simulink library "limblab"  (Simulink 8.0)
settings: Solver=ode45  SolverMode=SingleTasking  StartTime=0.0  StopTime=10.0  RelTol=1e-3
undefined symbols (not defined in the file or in its folder): dfilt, DiscIntNeverNeededParam
libraries: simulink x25, xpclib x10, limblab x9, xpcnilib x5, dsparch4 x4, dspsigops x2, xpcmeasurementcomputinglib x2, dspmtrx3 x1, simulink_extras x1
(part 1 of 2)
settings Model: Creator=limblab  LastModifiedBy=system administrator

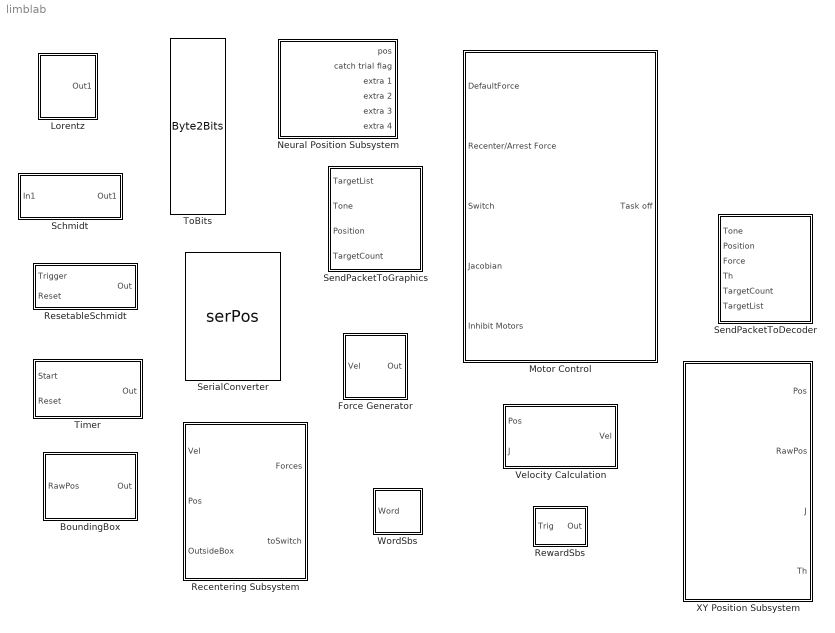
== system limblab ==
  BoundingBox : Subsystem
  Force Generator : Subsystem
  Lorentz : Subsystem  mask(Lorentz attractor){y0=.1}
      mask prompts: y0 "Initial Condition"
      mask help: Creats chaotic oscelations using a lorentz attractor algorithm.
      mask Help:
      | Creats chaotic oscelations using a lorentz attractor algorithm.
      | 
      | This particular oscilator has the parameters:
      | rho = 28
      | beta = 8/3
      | sigma = 10
      | 
      | The initial condition y0 can be specified as a parameter.
      | 
      | Other initial conditions (x0 and z0) are 0.1.
      mask Display: port_label('output', 1, 'Out')
  Motor Control : Subsystem
  Neural Position Subsystem : Subsystem  SystemSampleTime=0.01  mask(Neural Position Subsystem){}
      mask help: Uses a UDP receive block to receive and parse the sent neural position from the real time system.
      mask Display:
      | port_label('output',1,'pos')
      | port_label('output',2,'catch trial flag')
      | port_label('output',3,'extra 1')
      | port_label('output',4,'extra 2')
      | port_label('output',5,'extra 3')
      | port_label('output',6,'extra 4')
  Recentering Subsystem : Subsystem
  ResetableSchmidt : Subsystem  mask{Time=3}
  RewardSbs : Subsystem
  Schmidt : Subsystem  mask(Schmidt Trigger){Time=.3}
      mask help: Creates an output pulse of the specified time in seconds when trig goes high
      mask Help: Creates an output pulse of the specified time in seconds when trig goes high
      mask Display:
      | port_label('output',1,'out')
      | port_label('input',1,'trig')
      | fprintf('t = %.2f',Time)
  SendPacketToDecoder : Subsystem
  SendPacketToGraphics : Subsystem
  SerialConverter : S-Function  FunctionName=serPos  EnableBusSupport=off
      mask Display:
      | port_label('output', 1, 'Byte Out')
      | port_label('input', 1, 'index')
      | port_label('input', 2, 'sh')
      | port_label('input', 3, 'el')
  Timer : Subsystem  mask{Time=.1}
      mask prompts: Time "Timeout"
      mask Display:
      | port_label('output',1,'out')
      | port_label('input',1,'start')
      | port_label('input',2,'reset')
      | fprintf('t = %.2f',Time)
  ToBits : S-Function  FunctionName=Byte2Bits  EnableBusSupport=off
      mask Display:
      | port_label('input', 1, 'u')
      | port_label('output', 1, 'y0')
      | port_label('output', 2, 'y1')
      | port_label('output', 3, 'y2')
      | port_label('output', 4, 'y3')
      | port_label('output', 5, 'y4')
      | port_label('output', 6, 'y5')
      | port_label('output', 7, 'y6')
      | port_label('output', 8, 'y7')
  Velocity Calculation : Subsystem
  WordSbs : Subsystem
  XY Position Subsystem : Subsystem

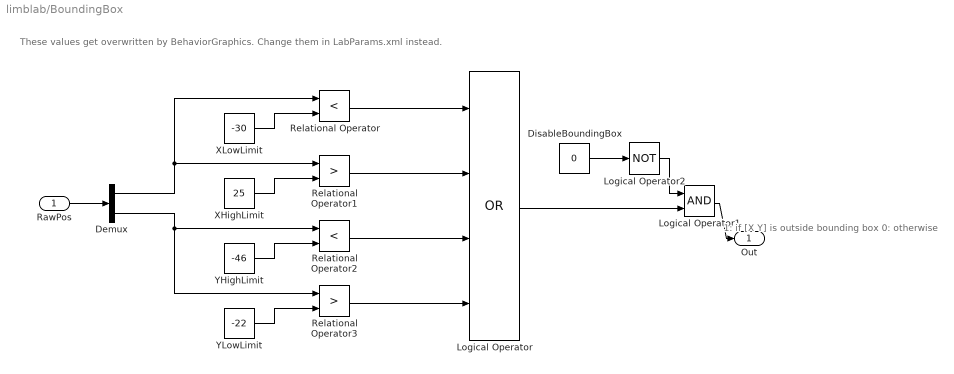
== system limblab/BoundingBox ==
  note: These values get overwritten by BehaviorGraphics. Change them in LabParams.xml instead.
  note: 1: if [X Y] is outside
      | bounding box
      | 0: otherwise
  RawPos : Inport
  Demux : Demux  Outputs=2
  DisableBoundingBox : Constant  Value=0
  Logical Operator : Logic  Operator=OR  Inputs=4  AllPortsSameDT=off  OutDataTypeStr=boolean
  Logical Operator1 : Logic  AllPortsSameDT=off  OutDataTypeStr=boolean
  Logical Operator2 : Logic  Operator=NOT  AllPortsSameDT=off  OutDataTypeStr=boolean
  Relational Operator : RelationalOperator  Operator=<  OutDataTypeStr=boolean
  Relational Operator1 : RelationalOperator  Operator=>  OutDataTypeStr=boolean
  Relational Operator2 : RelationalOperator  Operator=<  OutDataTypeStr=boolean
  Relational Operator3 : RelationalOperator  Operator=>  OutDataTypeStr=boolean
  XHighLimit : Constant  Value=25
  XLowLimit : Constant  Value=-30
  YHighLimit : Constant  Value=-46
  YLowLimit : Constant  Value=-22
  Out : Outport
  wires:
  XLowLimit/1 -> Relational Operator/2
  XHighLimit/1 -> Relational Operator1/2
  YHighLimit/1 -> Relational Operator2/2
  YLowLimit/1 -> Relational Operator3/2
  Relational Operator/1 -> Logical Operator/1
  Relational Operator1/1 -> Logical Operator/2
  Relational Operator2/1 -> Logical Operator/3
  Relational Operator3/1 -> Logical Operator/4
  RawPos/1 -> Demux/1
  Demux/1 -> Relational Operator/1, Relational Operator1/1
  Demux/2 -> Relational Operator2/1, Relational Operator3/1
  Logical Operator1/1 -> Out/1
  Logical Operator/1 -> Logical Operator1/2
  DisableBoundingBox/1 -> Logical Operator2/1
  Logical Operator2/1 -> Logical Operator1/1

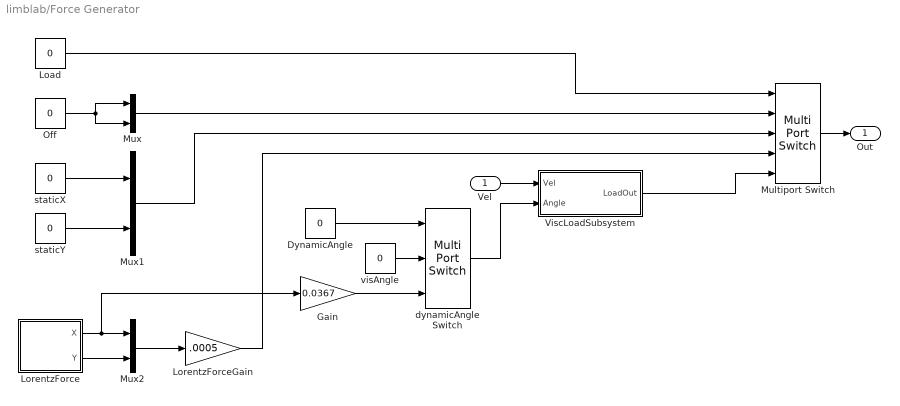
== system limblab/Force Generator ==
  Vel : Inport
  DynamicAngle : Constant  Value=0
  Gain : Gain  Gain=0.0367
  Load : Constant  Value=0
  LorentzForce : Subsystem
  LorentzForceGain : Gain  Gain=.0005
  Multiport Switch : MultiPortSwitch  DataPortOrder=Zero-based contiguous  Inputs=4  zeroidx=on
  Mux : Mux  Inputs=2
  Mux1 : Mux  Inputs=2
  Mux2 : Mux  Inputs=2
  Off : Constant  Value=0
  ViscLoadSubsystem : Subsystem
  dynamicAngle Switch : MultiPortSwitch  DataPortOrder=Zero-based contiguous  Inputs=2  zeroidx=on
  staticX : Constant  Value=0
  staticY : Constant  Value=0
  visAngle : Constant  Value=0
  Out : Outport
  wires:
  Off/1 -> Mux/2, Mux/1
  Multiport Switch/1 -> Out/1
  Mux/1 -> Multiport Switch/2
  Load/1 -> Multiport Switch/1
  Mux1/1 -> Multiport Switch/3
  staticX/1 -> Mux1/1
  staticY/1 -> Mux1/2
  LorentzForce/1(X) -> Mux2/1, Gain/1
  LorentzForce/2(Y) -> Mux2/2
  Mux2/1 -> LorentzForceGain/1
  LorentzForceGain/1 -> Multiport Switch/4
  Vel/1 -> ViscLoadSubsystem/1(Vel)
  ViscLoadSubsystem/1(LoadOut) -> Multiport Switch/5
  visAngle/1 -> dynamicAngle Switch/2
  DynamicAngle/1 -> dynamicAngle Switch/1
  dynamicAngle Switch/1 -> ViscLoadSubsystem/2(Angle)
  Gain/1 -> dynamicAngle Switch/3

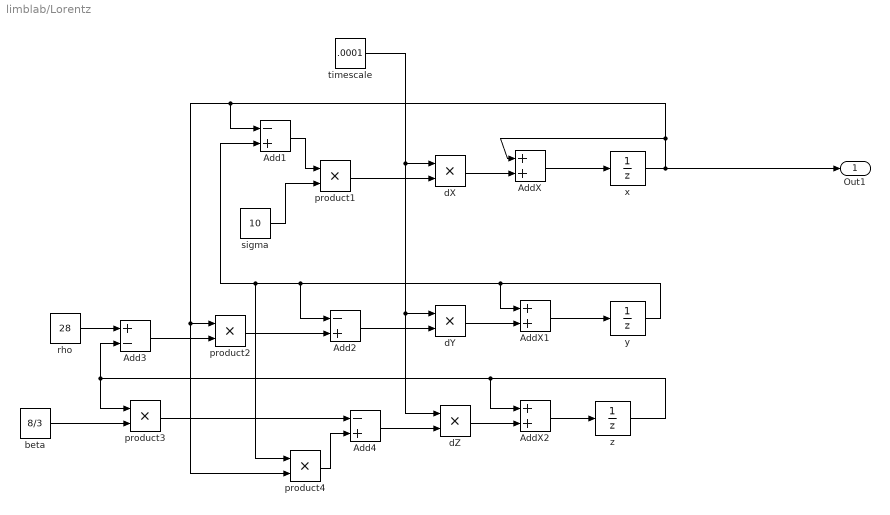
== system limblab/Lorentz ==
  Add1 : Sum  Inputs=-+
  Add2 : Sum  Inputs=-+
  Add3 : Sum  Inputs=+-
  Add4 : Sum  Inputs=-+
  AddX : Sum
  AddX1 : Sum
  AddX2 : Sum
  beta : Constant  Value=8/3
  dX : Product  RndMeth=Zero
  dY : Product  RndMeth=Zero
  dZ : Product  RndMeth=Zero
  product{1..4} (4 alike) : Product  RndMeth=Zero
  rho : Constant  Value=28
  sigma : Constant  Value=10
  timescale : Constant  Value=.0001
  x : UnitDelay  InitialCondition=.1  SampleTime=.001
  y : UnitDelay  InitialCondition=y0  SampleTime=.001
  z : UnitDelay  InitialCondition=.1  SampleTime=.001
  Out1 : Outport
  wires:
  AddX/1 -> x/1
  AddX1/1 -> y/1
  AddX2/1 -> z/1
  y/1 -> AddX1/1, Add2/1, Add1/2, product4/1
  z/1 -> AddX2/1, Add3/2, product3/1
  x/1 -> Out1/1, AddX/1, Add1/1, product2/1, product4/2
  dX/1 -> AddX/2
  dY/1 -> AddX1/2
  dZ/1 -> AddX2/2
  timescale/1 -> dX/1, dY/1, dZ/1
  sigma/1 -> product1/2
  product1/1 -> dX/2
  Add1/1 -> product1/1
  Add2/1 -> dY/2
  product2/1 -> Add2/2
  Add3/1 -> product2/2
  rho/1 -> Add3/1
  beta/1 -> product3/2
  product3/1 -> Add4/1
  product4/1 -> Add4/2
  Add4/1 -> dZ/2

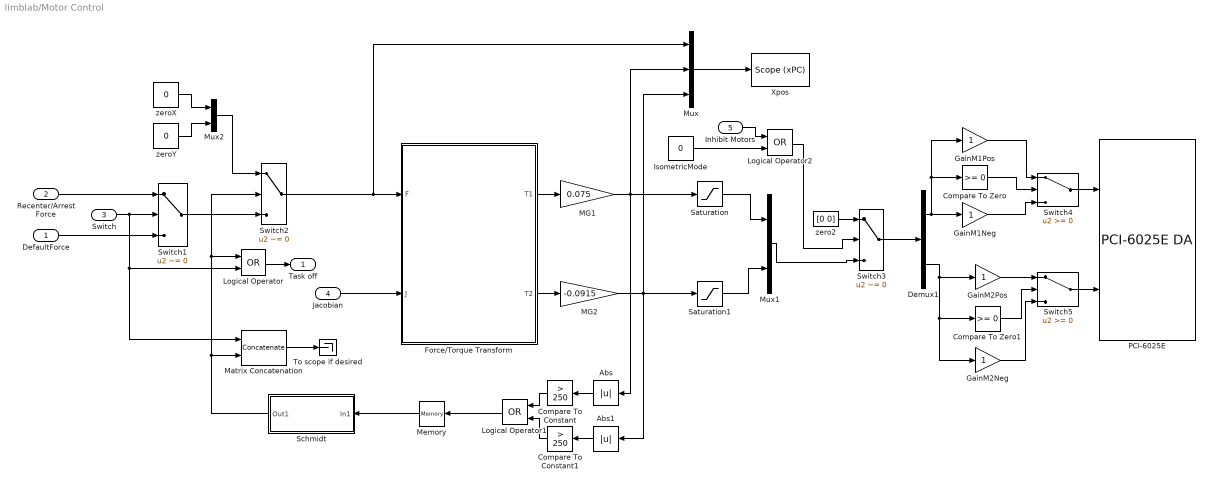
== system limblab/Motor Control ==
  DefaultForce : Inport
  Recenter/Arrest Force : Inport  Port=2
  Switch : Inport  Port=3
  Jacobian : Inport  Port=4
  Inhibit Motors : Inport  Port=5
  Abs : Abs
  Abs1 : Abs
  Compare To Constant : simulink/Logic and Bit Operations/Compare To Constant  relop=>  const=250  OutDataTypeStr=uint8  ZeroCross=off
  Compare To Constant1 : simulink/Logic and Bit Operations/Compare To Constant  relop=>  const=250  OutDataTypeStr=uint8  ZeroCross=off
  Compare To Zero : simulink/Logic and Bit Operations/Compare To Zero  relop=>=  OutDataTypeStr=boolean
  Compare To Zero1 : simulink/Logic and Bit Operations/Compare To Zero  relop=>=  OutDataTypeStr=boolean
  Demux1 : Demux  Outputs=2
  Force/Torque Transform : Subsystem  TreatAsAtomicUnit=on
  GainM1Neg : Gain
  GainM1Pos : Gain
  GainM2Neg : Gain
  GainM2Pos : Gain
  IsometricMode : Constant  Value=0
  Logical Operator1 : Logic  Operator=OR  AllPortsSameDT=off  OutDataTypeStr=boolean
  Logical Operator : Logic  Operator=OR  AllPortsSameDT=off  OutDataTypeStr=boolean
  Logical Operator2 : Logic  Operator=OR  AllPortsSameDT=off  OutDataTypeStr=boolean
  MG1 : Gain  Gain=0.075
  MG2 : Gain  Gain=-0.0915
  Matrix Concatenation : Concatenate
  Memory : Memory
  Mux : Mux  Inputs=3
  Mux1 : Mux  Inputs=2
  Mux2 : Mux  Inputs=2
  "PCI-6025E " : xpcnilib/D//A/E Series/PCI-6025E DA  channel=[1 2]  reset=[1 1]  initValue=[0 0]  sampletime=0.001  slot=-1
  Saturation : Saturate  UpperLimit=7.5  LowerLimit=-7.5
  Saturation1 : Saturate  UpperLimit=7.5  LowerLimit=-7.5
  Schmidt : Subsystem  mask(Schmidt Trigger){Time=10}
      mask help: Creates an output pulse of the specified time in seconds when trig goes high
      mask Help: Creates an output pulse of the specified time in seconds when trig goes high
      mask Display:
      | port_label('output',1,'out')
      | port_label('input',1,'trig')
      | fprintf('t = %d',Time)
  Switch1 : Switch  Criteria=u2 ~= 0  ZeroCross=off
  Switch2 : Switch  Criteria=u2 ~= 0  ZeroCross=off
  Switch3 : Switch  Criteria=u2 ~= 0  ZeroCross=off
  Switch4 : Switch
  Switch5 : Switch
  To scope if desired : Terminator
  Xpos : xpclib/Misc./Scope (xPC)   scopeno=4  scopetype=Target  autostart=on  viewmode=Numerical  formatstr='%15.2f Fx,%15.2f Fy,%15.2f T1,%15.2f T2'  grid=on  ylimits=[-10,10]  nosamples=10  noprepostsamples=0  interleave=10  triggermode=FreeRun  triggersignal=1  triggerlevel=0.0  triggerslope=Either  triggerscope=1  triggersample=0  filename=data.dat  mode=Lazy  writesize=512  autorestart=off  dynamicfilemode=off  maxwritefilesize=512*1024^2
  zero2 : Constant  Value=[0 0]
  zeroX : Constant  Value=0
  zeroY : Constant  Value=0
  Task off : Outport
  wires:
  MG1/1 -> Abs/1, Saturation/1, Mux/2
  MG2/1 -> Abs1/1, Saturation1/1, Mux/3
  Force/Torque Transform/1(T1) -> MG1/1
  Force/Torque Transform/2(T2) -> MG2/1
  zeroX/1 -> Mux2/1
  zeroY/1 -> Mux2/2
  Mux2/1 -> Switch2/1
  Switch1/1 -> Switch2/3
  Switch2/1 -> Force/Torque Transform/1(F), Mux/1
  Schmidt/1(Out1) -> Logical Operator/1, Switch2/2, Matrix Concatenation/2
  Compare To Constant/1 -> Logical Operator1/1
  Compare To Constant1/1 -> Logical Operator1/2
  Memory/1 -> Schmidt/1(In1)
  Logical Operator1/1 -> Memory/1
  Matrix Concatenation/1 -> To scope if desired/1
  Jacobian/1 -> Force/Torque Transform/2(J)
  Switch/1 -> Switch1/2, Logical Operator/2, Matrix Concatenation/1
  DefaultForce/1 -> Switch1/3
  Recenter/Arrest Force/1 -> Switch1/1
  Mux/1 -> Xpos/1
  Logical Operator/1 -> Task off/1
  Saturation/1 -> Mux1/1
  Saturation1/1 -> Mux1/2
  zero2/1 -> Switch3/1
  Mux1/1 -> Switch3/3
  Switch3/1 -> Demux1/1
  Demux1/1 -> GainM1Pos/1, Compare To Zero/1, GainM1Neg/1
  Abs/1 -> Compare To Constant/1
  Abs1/1 -> Compare To Constant1/1
  Compare To Zero/1 -> Switch4/2
  GainM1Pos/1 -> Switch4/1
  Switch4/1 -> "PCI-6025E "/1
  GainM1Neg/1 -> Switch4/3
  Compare To Zero1/1 -> Switch5/2
  GainM2Pos/1 -> Switch5/1
  GainM2Neg/1 -> Switch5/3
  Switch5/1 -> "PCI-6025E "/2
  Demux1/2 -> GainM2Pos/1, GainM2Neg/1, Compare To Zero1/1
  Inhibit Motors/1 -> Logical Operator2/1
  Logical Operator2/1 -> Switch3/2
  IsometricMode/1 -> Logical Operator2/2

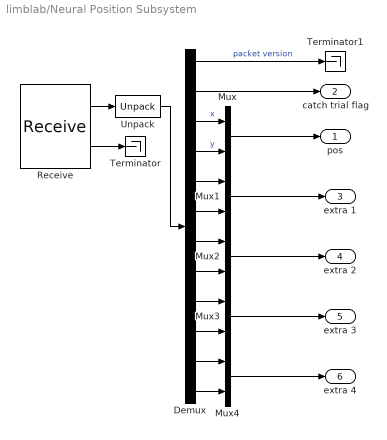
== system limblab/Neural Position Subsystem ==
  Demux : Demux  Outputs=12
  Mux{,1..4} (5 alike) : Mux  Inputs=2
  Receive : xpclib/UDP/Receive  ipAddress=0.0.0.0  ipPort=24999  width=48  vblLen=on  sampletime=0.001
  Terminator : Terminator
  Terminator1 : Terminator
  Unpack : xpclib/UDP/Unpack  dimensions={[1,12]}  datatypes={'single'}  byteAlign=1
  pos : Outport
  catch trial flag : Outport  Port=2
  extra 1 : Outport  Port=3
  extra 2 : Outport  Port=4
  extra 3 : Outport  Port=5
  extra 4 : Outport  Port=6
  wires:
  Demux/2 -> catch trial flag/1
  Mux/1 -> pos/1
  Demux/4 -> Mux/2  "y"
  Demux/3 -> Mux/1  "x"
  Demux/1 -> Terminator1/1  "packet version"
  Unpack/1 -> Demux/1
  Receive/2 -> Terminator/1
  Receive/1 -> Unpack/1
  Demux/5 -> Mux1/1
  Demux/6 -> Mux1/2
  Demux/7 -> Mux2/1
  Demux/8 -> Mux2/2
  Mux1/1 -> extra 1/1
  Mux2/1 -> extra 2/1
  Demux/9 -> Mux3/1
  Demux/10 -> Mux3/2
  Mux3/1 -> extra 3/1
  Demux/11 -> Mux4/1
  Demux/12 -> Mux4/2
  Mux4/1 -> extra 4/1

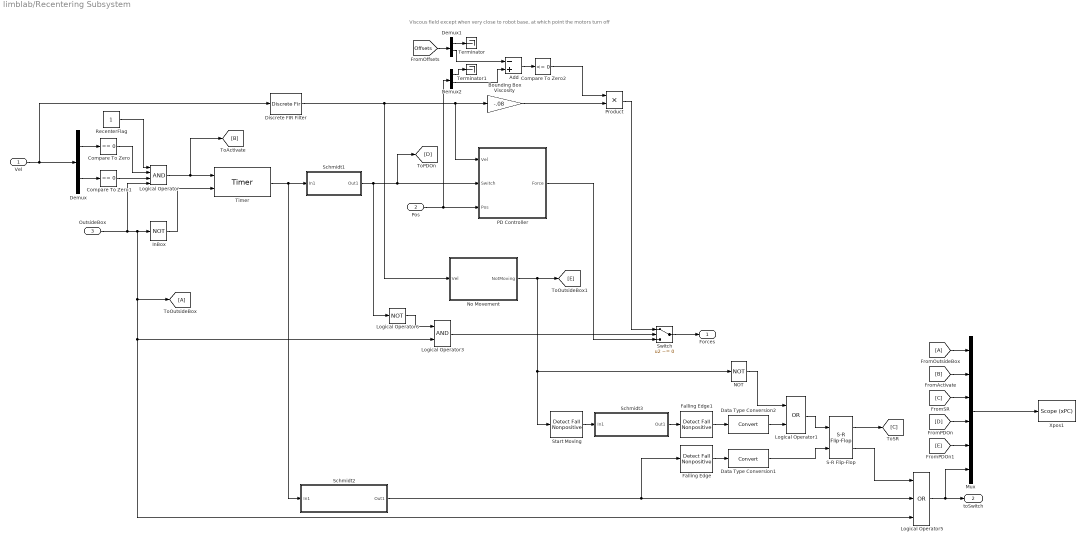
== system limblab/Recentering Subsystem ==
  note: Viscous field except when very close to robot base, at which point the motors turn off
  Vel : Inport
  Pos : Inport  Port=2
  OutsideBox : Inport  Port=3
  Add : Sum  Inputs=-+
  Bounding Box Viscosity : Gain  Gain=-.08
  Compare To Zero : simulink/Logic and Bit Operations/Compare To Zero  relop===  OutDataTypeStr=uint8  ZeroCross=off
  Compare To Zero1 : simulink/Logic and Bit Operations/Compare To Zero  relop===  OutDataTypeStr=uint8  ZeroCross=off
  Compare To Zero2 : simulink/Logic and Bit Operations/Compare To Zero  relop=<=  OutDataTypeStr=boolean
  Data Type Conversion1 : DataTypeConversion
  Data Type Conversion2 : DataTypeConversion
  Demux : Demux  Outputs=2
  Demux1 : Demux  Outputs=2
  Demux2 : Demux  Outputs=2
  Discrete FIR Filter : DiscreteFir  Coefficients="[0.0069    0.0195    0.0106    0.0194    0.0217    0.0270    0.0313    0.0360    0.0404    0.0445    0.0482    0.0513    0.0538    0.0554    0.0563    0.0563    0.0554 0.0538    0.0513    0.0482    0.0445    0.0404    0.0360    0.0313    0.0270    0.0217    0.0194    0.0106    0.0195    0.0069]"
  Falling Edge : simulink/Logic and Bit Operations/Detect Fall Nonpositive  vinit=0  InputProcessing=Inherited  OutDataTypeStr=uint8
  Falling Edge1 : simulink/Logic and Bit Operations/Detect Fall Nonpositive  vinit=0  InputProcessing=Inherited  OutDataTypeStr=uint8
  InBox : Logic  Operator=NOT  AllPortsSameDT=off  OutDataTypeStr=boolean
  Logical Operator : Logic  Inputs=4  AllPortsSameDT=off  OutDataTypeStr=boolean
  Logical Operator1 : Logic  Operator=OR  AllPortsSameDT=off  OutDataTypeStr=boolean
  Logical Operator3 : Logic  AllPortsSameDT=off  OutDataTypeStr=boolean
  Logical Operator5 : Logic  Operator=OR  Inputs=3  AllPortsSameDT=off  OutDataTypeStr=boolean
  Logical Operator6 : Logic  Operator=NOT  AllPortsSameDT=off  OutDataTypeStr=boolean
  Mux : Mux  Inputs=6
  NOT : Logic  Operator=NOT  AllPortsSameDT=off  OutDataTypeStr=boolean
  No Movement : Subsystem
  PD Controller : Subsystem
  Product : Product  RndMeth=Zero
  RecenterFlag : Constant
  S-R Flip-Flop : simulink_extras/Flip Flops/S-R Flip-Flop  initial_condition=0
  Schmidt1 : Subsystem  mask(Schmidt Trigger){Time=4}
      mask help: Creates an output pulse of the specified time in seconds when trig goes high
      mask Help: Creates an output pulse of the specified time in seconds when trig goes high
      mask Display:
      | port_label('output',1,'out')
      | port_label('input',1,'trig')
      | fprintf('t = %d',Time)
  Schmidt2 : Subsystem  mask(Schmidt Trigger){Time=5}
      mask help: Creates an output pulse of the specified time in seconds when trig goes high
      mask Help: Creates an output pulse of the specified time in seconds when trig goes high
      mask Display:
      | port_label('output',1,'out')
      | port_label('input',1,'trig')
      | fprintf('t = %d',Time)
  Schmidt3 : Subsystem  mask(Schmidt Trigger){Time=0.5}
      mask help: Creates an output pulse of the specified time in seconds when trig goes high
      mask Help: Creates an output pulse of the specified time in seconds when trig goes high
      mask Display:
      | port_label('output',1,'out')
      | port_label('input',1,'trig')
      | fprintf('t = %d',Time)
  Start Moving : simulink/Logic and Bit Operations/Detect Fall Nonpositive  vinit=0  InputProcessing=Inherited  OutDataTypeStr=uint8
  Switch : Switch  Criteria=u2 ~= 0
  Terminator : Terminator
  Terminator1 : Terminator
  Timer : limblab/Timer  Time=10
  Xpos1 : xpclib/Misc./Scope (xPC)   scopeno=2  scopetype=Target  autostart=on  viewmode=Numerical  formatstr='%2.0f OutsideBox,%2.0f Activate,%2.0f SR,%2.0f OD On,%2.0f no movement,%2.0f claimed'  grid=on  ylimits=[-10,10]  nosamples=10  noprepostsamples=0  interleave=10  triggermode=FreeRun  triggersignal=1  triggerlevel=0.0  triggerslope=Either  triggerscope=1  triggersample=0  filename=data.dat  mode=Lazy  writesize=512  autorestart=off  dynamicfilemode=off  maxwritefilesize=512*1024^2
  Forces : Outport
  toSwitch : Outport  Port=2
  wires:
  Demux/2 -> Compare To Zero1/1
  Compare To Zero/1 -> Logical Operator/2
  Schmidt1/1(Out1) -> Logical Operator6/1, PD Controller/2(Switch), [D]
  Logical Operator/1 -> Timer/1, [B]
  OutsideBox/1 -> [A], Logical Operator3/2, Logical Operator5/3, InBox/1, Logical Operator/4
  Switch/1 -> Forces/1
  Logical Operator5/1 -> toSwitch/1, Mux/6
  Logical Operator6/1 -> Logical Operator3/1
  InBox/1 -> Timer/2
  Vel/1 -> Demux/1, Discrete FIR Filter/1
  Timer/1 -> Schmidt1/1(In1), Schmidt2/1(In1)
  Compare To Zero1/1 -> Logical Operator/3
  Demux/1 -> Compare To Zero/1
  Logical Operator3/1 -> Switch/2
  RecenterFlag/1 -> Logical Operator/1
  PD Controller/1(Force) -> Switch/3
  Pos/1 -> Demux2/1, PD Controller/3(Pos)
  Bounding Box Viscosity/1 -> Product/2
  Mux/1 -> Xpos1/1
  [A] -> Mux/1
  [B] -> Mux/2
  [D] -> Mux/4
  [C] -> Mux/3
  [E] -> Mux/5
  Schmidt2/1(Out1) -> Logical Operator5/2, Falling Edge/1
  S-R Flip-Flop/1 -> [C]
  S-R Flip-Flop/2 -> Logical Operator5/1
  Falling Edge/1 -> Data Type Conversion1/1
  Data Type Conversion1/1 -> S-R Flip-Flop/2
  Start Moving/1 -> Schmidt3/1(In1)
  Schmidt3/1(Out1) -> Falling Edge1/1
  Falling Edge1/1 -> Data Type Conversion2/1
  Data Type Conversion2/1 -> Logical Operator1/2
  Logical Operator1/1 -> S-R Flip-Flop/1
  No Movement/1(NotMoving) -> [E], Start Moving/1, NOT/1
  NOT/1 -> Logical Operator1/1
  [Offsets] -> Demux1/1
  Demux1/1 -> Terminator/1
  Demux2/1 -> Terminator1/1
  Demux1/2 -> Add/1
  Demux2/2 -> Add/2
  Add/1 -> Compare To Zero2/1
  Compare To Zero2/1 -> Product/1
  Product/1 -> Switch/1
  Discrete FIR Filter/1 -> No Movement/1(Vel), PD Controller/1(Vel), Bounding Box Viscosity/1

== system limblab/ResetableSchmidt ==
  Trigger : Inport
  Reset : Inport  Port=2
  Clock : Clock
  Compare To Zero : simulink/Logic and Bit Operations/Compare To Zero  relop=>  OutDataTypeStr=uint8  ZeroCross=off
  Enabled Subsystem : Subsystem  TreatAsAtomicUnit=on
  Logical Operator : Logic  Operator=XOR  AllPortsSameDT=off  OutDataTypeStr=boolean  SampleTime=.001
  Logical Operator1 : Logic  Operator=NOT  AllPortsSameDT=off  OutDataTypeStr=boolean
  Logical Operator2 : Logic  Operator=OR  AllPortsSameDT=off  OutDataTypeStr=boolean  SampleTime=.001
  Logical Operator3 : Logic  Operator=NOT  AllPortsSameDT=off  OutDataTypeStr=boolean
  Logical Operator4 : Logic  AllPortsSameDT=off  OutDataTypeStr=boolean  SampleTime=.001
  Memory : Memory
  Relational Operator : RelationalOperator  Operator=>  OutDataTypeStr=boolean
  Sum : Sum  Inputs=-+
  Time : Constant  Value=Time
  Out : Outport
  wires:
  Logical Operator2/1 -> Logical Operator1/1
  Trigger/1 -> Logical Operator2/2
  Logical Operator/1 -> Memory/1, Out/1
  Logical Operator1/1 -> Enabled Subsystem/Enable
  Relational Operator/1 -> Logical Operator/2
  Compare To Zero/1 -> Logical Operator/1
  Time/1 -> Relational Operator/2
  Sum/1 -> Relational Operator/1, Compare To Zero/1
  Enabled Subsystem/1(Out1) -> Sum/1
  Clock/1 -> Sum/2, Enabled Subsystem/1(In1)
  Reset/1 -> Logical Operator3/1
  Logical Operator3/1 -> Logical Operator4/2
  Logical Operator4/1 -> Logical Operator2/1
  Memory/1 -> Logical Operator4/1

== system limblab/RewardSbs ==
  Trig : Inport
  Data Type Conversion : DataTypeConversion
  JackpotChance : Constant  Value=0
  Relational Operator : RelationalOperator  Operator=>  OutDataTypeStr=boolean
  RewardJackpot : Constant  Value=0.60
  RewardTime : Constant  Value=0.30
  Sample and Hold : dspsigops/Sample and Hold  trig=Rising edge  initCond=0  latchinput=off
  Schmidt : Subsystem
  Switch : Switch  Criteria=u2 > Threshold  ZeroCross=off
  Uniform Random Number : UniformRandomNumber  Minimum=0  Maximum=100  SampleTime=0.001
  Out : Outport
  wires:
  Trig/1 -> Schmidt/1(Trigger), Sample and Hold/Trigger
  Data Type Conversion/1 -> Out/1
  Schmidt/1(Output) -> Data Type Conversion/1
  Sample and Hold/1 -> Schmidt/2(Duration)
  RewardJackpot/1 -> Switch/3
  Switch/1 -> Sample and Hold/1
  Uniform Random Number/1 -> Relational Operator/1
  Relational Operator/1 -> Switch/2
  JackpotChance/1 -> Relational Operator/2
  RewardTime/1 -> Switch/1

== system limblab/Schmidt ==
  In1 : Inport
  Clock : Clock
  Compare To Zero : simulink/Logic and Bit Operations/Compare To Zero  relop=>  OutDataTypeStr=uint8  ZeroCross=off
  Enabled Subsystem : Subsystem  TreatAsAtomicUnit=on
  Logical Operator : Logic  Operator=XOR  AllPortsSameDT=off  OutDataTypeStr=boolean  SampleTime=.001
  Logical Operator1 : Logic  Operator=NOT  AllPortsSameDT=off  OutDataTypeStr=boolean
  Logical Operator2 : Logic  Operator=OR  AllPortsSameDT=off  OutDataTypeStr=boolean  SampleTime=.001
  Memory : Memory
  Relational Operator : RelationalOperator  Operator=>  OutDataTypeStr=boolean
  Sum : Sum  Inputs=-+
  Time : Constant  Value=Time
  Out1 : Outport
  wires:
  Clock/1 -> Enabled Subsystem/1(In1), Sum/2
  Enabled Subsystem/1(Out1) -> Sum/1
  Sum/1 -> Compare To Zero/1, Relational Operator/1
  Time/1 -> Relational Operator/2
  Compare To Zero/1 -> Logical Operator/1
  Relational Operator/1 -> Logical Operator/2
  Logical Operator1/1 -> Enabled Subsystem/Enable
  Logical Operator/1 -> Out1/1, Memory/1
  In1/1 -> Logical Operator2/2
  Logical Operator2/1 -> Logical Operator1/1
  Memory/1 -> Logical Operator2/1

== system limblab/SendPacketToDecoder ==
  note: This subsystem packs the information
      | to be sent to the Graphics Client.  The
      | Packet Spec tells the Graphics Client
      | how to parse the information.  The
      | original specification didn't send a version
      | number; it simply sent 16 doubles.  To
      | differentiate the two, I ensure the first
      | double is NaN.  The packet spec is then
      | parsed from inside the NaN's payload.
  note: The UDP sends its packets every other cycle
      | to a specific IP address and port.  It is not
      | broadcast.
      |
      | The TargetList is a stacked array
      | of 5 doubles repeated TargetCount times:
      | The TargetType, the upperleft X,Y position
      | and the lower right X, Y position.
  Tone : Inport  PortDimensions=[2]
  Position : Inport  Port=2  PortDimensions=[2]
  Force : Inport  Port=3
  Th : Inport  Port=4
  TargetCount : Inport  Port=5  PortDimensions=[1]
  TargetList : Inport  Port=6
  Demux{,1..3} (4 alike) : Demux  Outputs=2
  NaN upper bytes : Constant  Value=hex2dec('fff80000')  OutDataTypeStr=uint32
  Pack : xpclib/UDP/Pack  datatypes={'uint32','uint32','double','double','double','double','double','double','double','double','double','double'}  byteAlign=1
  Packet Spec : Constant  OutDataTypeStr=uint32
  Rate Transition : RateTransition
  Send : xpclib/UDP/Send  ipAddress=192.168.0.10  ipPort=24998  localPort=-1  vblLen=off  sampletime=.001
  wires:
  Rate Transition/1 -> Send/1
  Pack/1 -> Rate Transition/1
  Tone/1 -> Demux/1
  Position/1 -> Demux1/1
  Demux1/2 -> Pack/6
  Demux1/1 -> Pack/5
  Demux/2 -> Pack/4
  Demux/1 -> Pack/3
  NaN upper bytes/1 -> Pack/2
  Packet Spec/1 -> Pack/1
  Force/1 -> Demux2/1
  Demux2/1 -> Pack/7
  Demux2/2 -> Pack/8
  Th/1 -> Demux3/1
  Demux3/1 -> Pack/9
  Demux3/2 -> Pack/10
  TargetCount/1 -> Pack/11
  TargetList/1 -> Pack/12

== system limblab/SendPacketToGraphics ==
  note: This subsystem packs the information
      | to be sent to the Graphics Client.  The
      | Packet Spec tells the Graphics Client
      | how to parse the information.  The
      | original specification didn't send a version
      | number; it simply sent 16 doubles.  To
      | differentiate the two, I ensure the first
      | double is NaN.  The packet spec is then
      | parsed from inside the NaN's payload.
  note: The UDP sends its packets every other cycle
      | to a specific IP address and port.  It is not
      | broadcast.
      |
      | The TargetList is a stacked array
      | of 5 doubles repeated TargetCount times:
      | The TargetType, the upperleft X,Y position
      | and the lower right X, Y position.
  TargetList : Inport
  Tone : Inport  Port=2  PortDimensions=[2]
  Position : Inport  Port=3  PortDimensions=[2]
  TargetCount : Inport  Port=4  PortDimensions=[1]
  Demux : Demux  Outputs=2
  Demux1 : Demux  Outputs=2
  NaN upper bytes : Constant  Value=hex2dec('fff80000')  OutDataTypeStr=uint32
  Pack : xpclib/UDP/Pack  datatypes={'uint32','uint32','double','double','double','double','double','double'}  byteAlign=1
  Packet Spec : Constant  OutDataTypeStr=uint32
  Rate Transition : RateTransition
  Send : xpclib/UDP/Send  ipAddress=192.168.0.2  ipPort=25000  localPort=-1  vblLen=off  sampletime=.02
  wires:
  Rate Transition/1 -> Send/1
  Pack/1 -> Rate Transition/1
  Tone/1 -> Demux/1
  Position/1 -> Demux1/1
  TargetList/1 -> Pack/8
  TargetCount/1 -> Pack/7
  Demux1/2 -> Pack/6
  Demux1/1 -> Pack/5
  Demux/2 -> Pack/4
  Demux/1 -> Pack/3
  NaN upper bytes/1 -> Pack/2
  Packet Spec/1 -> Pack/1

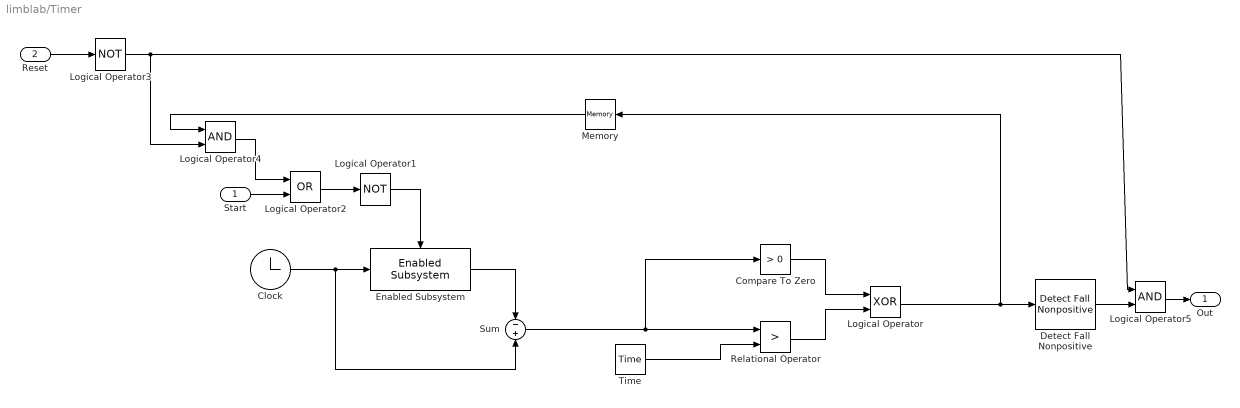
== system limblab/Timer ==
  Start : Inport
  Reset : Inport  Port=2
  Clock : Clock
  Compare To Zero : simulink/Logic and Bit Operations/Compare To Zero  relop=>  OutDataTypeStr=uint8  ZeroCross=off
  Detect Fall Nonpositive : simulink/Logic and Bit Operations/Detect Fall Nonpositive  vinit=0  InputProcessing=Inherited  OutDataTypeStr=uint8
  Enabled Subsystem : limblab/ResetableSchmidt/Enabled Subsystem
  Logical Operator : Logic  Operator=XOR  AllPortsSameDT=off  OutDataTypeStr=boolean  SampleTime=.001
  Logical Operator1 : Logic  Operator=NOT  AllPortsSameDT=off  OutDataTypeStr=boolean
  Logical Operator2 : Logic  Operator=OR  AllPortsSameDT=off  OutDataTypeStr=boolean  SampleTime=.001
  Logical Operator3 : Logic  Operator=NOT  AllPortsSameDT=off  OutDataTypeStr=boolean
  Logical Operator4 : Logic  AllPortsSameDT=off  OutDataTypeStr=boolean  SampleTime=.001
  Logical Operator5 : Logic  AllPortsSameDT=off  OutDataTypeStr=boolean  SampleTime=.001
  Memory : Memory
  Relational Operator : RelationalOperator  Operator=>  OutDataTypeStr=boolean
  Sum : Sum  Inputs=-+
  Time : Constant  Value=Time
  Out : Outport
  wires:
  Memory/1 -> Logical Operator4/1
  Logical Operator4/1 -> Logical Operator2/1
  Logical Operator3/1 -> Logical Operator5/1, Logical Operator4/2
  Reset/1 -> Logical Operator3/1
  Clock/1 -> Sum/2, Enabled Subsystem/1
  Enabled Subsystem/1 -> Sum/1
  Sum/1 -> Relational Operator/1, Compare To Zero/1
  Time/1 -> Relational Operator/2
  Compare To Zero/1 -> Logical Operator/1
  Relational Operator/1 -> Logical Operator/2
  Logical Operator1/1 -> Enabled Subsystem/Enable
  Logical Operator/1 -> Memory/1, Detect Fall Nonpositive/1
  Start/1 -> Logical Operator2/2
  Logical Operator2/1 -> Logical Operator1/1
  Detect Fall Nonpositive/1 -> Logical Operator5/2
  Logical Operator5/1 -> Out/1

== system limblab/Velocity Calculation ==
  Pos : Inport
  J : Inport  Port=2
  Demux : Demux  Outputs=2
  Matrix Multiply : Product  Multiplication=Matrix(*)
  Mux1 : Mux  Inputs=2
  Mux2 : Mux  Inputs=2
  Pos2VelX : Subsystem
  Pos2VelY : Subsystem
  ReplaceIfYouWantToUseTachs1 : Constant  Value=0
  ReplaceIfYouWantToUseTachs2 : Constant  Value=0
  Switch : Switch  Threshold=.5
  TachGain1 : Gain  Gain=1.29
  TachGain2 : Gain  Gain=1.29
  UseTachs : Constant  Value=0
  Vel : Outport
  wires:
  Pos2VelX/1(Out) -> Mux1/1
  Pos2VelY/1(Out) -> Mux1/2
  Demux/1 -> Pos2VelX/1(In)
  Demux/2 -> Pos2VelY/1(In)
  Pos/1 -> Demux/1
  UseTachs/1 -> Switch/2
  ReplaceIfYouWantToUseTachs1/1 -> TachGain1/1
  ReplaceIfYouWantToUseTachs2/1 -> TachGain2/1
  TachGain1/1 -> Mux2/1
  TachGain2/1 -> Mux2/2
  J/1 -> Matrix Multiply/1
  Mux2/1 -> Matrix Multiply/2
  Switch/1 -> Vel/1
  Mux1/1 -> Switch/3
  Matrix Multiply/1 -> Switch/1

== system limblab/WordSbs ==
  Word : Inport
  tag scope: Word=global
  wires:
  Word/1 -> [Word]

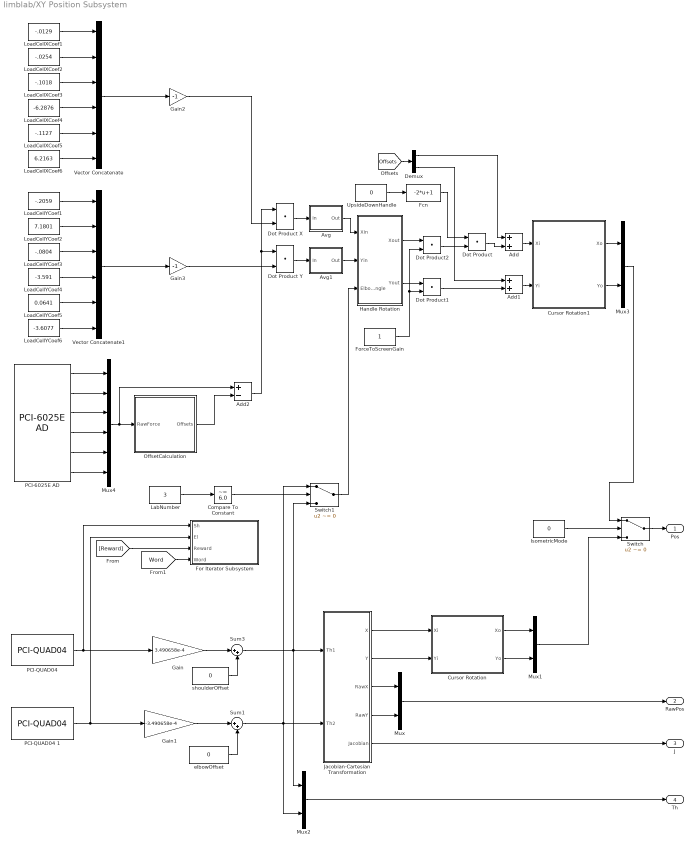
== system limblab/XY Position Subsystem ==
  Add : Sum
  Add1 : Sum
  Add2 : Sum  Inputs=+-
  Avg : Subsystem
  Avg1 : Subsystem
  Compare To Constant : simulink/Logic and Bit Operations/Compare To Constant  relop=~=  const=6.0  OutDataTypeStr=boolean
  Cursor Rotation : Subsystem
  Cursor Rotation1 : Subsystem
  Demux : Demux  Outputs=2
  Dot Product : DotProduct  InputSameDT=on  OutDataTypeStr=Inherit: Inherit via internal rule
  Dot Product X : DotProduct  InputSameDT=on  OutDataTypeStr=Inherit: Inherit via internal rule
  Dot Product Y : DotProduct  InputSameDT=on  OutDataTypeStr=Inherit: Inherit via internal rule
  Dot Product1 : DotProduct  InputSameDT=on  OutDataTypeStr=Inherit: Inherit via internal rule
  Dot Product2 : DotProduct  InputSameDT=on  OutDataTypeStr=Inherit: Inherit via internal rule
  Fcn : Fcn  Expr=-2*u+1
  For Iterator Subsystem : Subsystem  TreatAsAtomicUnit=on
  ForceToScreenGain : Constant
  Gain : Gain  Gain=3.490658e-4
  Gain1 : Gain  Gain=-3.490658e-4
  Gain2 : Gain  Gain=-1
  Gain3 : Gain  Gain=-1
  Handle Rotation : Subsystem
  IsometricMode : Constant  Value=0
  Jacobian-Cartesian Transformation : Subsystem
  LabNumber : Constant  Value=3
  LoadCellXCoef1 : Constant  Value=-.0129
  LoadCellXCoef2 : Constant  Value=-.0254
  LoadCellXCoef3 : Constant  Value=-.1018
  LoadCellXCoef4 : Constant  Value=-6.2876
  LoadCellXCoef5 : Constant  Value=-.1127
  LoadCellXCoef6 : Constant  Value=6.2163
  LoadCellYCoef1 : Constant  Value=-.2059
  LoadCellYCoef2 : Constant  Value=7.1801
  LoadCellYCoef3 : Constant  Value=-.0804
  LoadCellYCoef4 : Constant  Value=-3.591
  LoadCellYCoef5 : Constant  Value=0.0641
  LoadCellYCoef6 : Constant  Value=-3.6077
  Mux{,1..3} (4 alike) : Mux  Inputs=2
  Mux4 : Mux  Inputs=6
  OffsetCalculation : Subsystem
  PCI-6025E AD : xpcnilib/A//D/E Series/PCI-6025E AD  channel=[11 12 13 14 15 16]  range=[-10 -10 -10 -10 -10 -10]  coupling=[0 0 0 0 0 0]  sampletime=0.001  slot=-1
  "PCI-QUAD04 " : xpcmeasurementcomputinglib/Incremental Encoder/PCI-QUAD04   channel=1  resetmode=on  polarity=Positive Index  mode=Normal  limit=0  range=-2^23...+2^23-1  speed=1x  prescale=0  ts=0.001  convbaseaddr=-1
  PCI-QUAD04 1 : xpcmeasurementcomputinglib/Incremental Encoder/PCI-QUAD04   channel=2  resetmode=on  polarity=Positive Index  mode=Normal  limit=0  range=-2^23...+2^23-1  speed=1x  prescale=0  ts=0.001  convbaseaddr=-1
  Sum1 : Sum  Inputs=|++  SaturateOnIntegerOverflow=on  InputSameDT=on  OutDataTypeStr=Inherit: Same as first input
  Sum3 : Sum  Inputs=|++  SaturateOnIntegerOverflow=on  InputSameDT=on  OutDataTypeStr=Inherit: Same as first input
  Switch : Switch  Criteria=u2 ~= 0
  Switch1 : Switch  Criteria=u2 ~= 0
  UpsideDownHandle : Constant  Value=0
  Vector Concatenate : Concatenate  NumInputs=6  Mode=Multidimensional array  ConcatenateDimension=2
  Vector Concatenate1 : Concatenate  NumInputs=6  Mode=Multidimensional array  ConcatenateDimension=2
  elbowOffset : Constant  Value=0
  shoulderOffset : Constant  Value=0
  Pos : Outport
  RawPos : Outport  Port=2
  J : Outport  Port=3
  Th : Outport  Port=4
  wires:
  PCI-QUAD04 1/1 -> Gain1/1, For Iterator Subsystem/2("El ")
  "PCI-QUAD04 "/1 -> For Iterator Subsystem/1(Sh), Gain/1
  Gain/1 -> Sum3/1
  Sum3/1 -> Switch1/3, Mux2/1, Jacobian-Cartesian Transformation/1(Th1)
  shoulderOffset/1 -> Sum3/2
  Gain1/1 -> Sum1/1
  elbowOffset/1 -> Sum1/2
  Sum1/1 -> Switch1/1, Mux2/2, Jacobian-Cartesian Transformation/2(Th2)
  Jacobian-Cartesian Transformation/1(X) -> Cursor Rotation/1(Xi)
  Jacobian-Cartesian Transformation/2(Y) -> Cursor Rotation/2(Yi)
  Cursor Rotation/1(Xo) -> Mux1/1
  Cursor Rotation/2(Yo) -> Mux1/2
  Jacobian-Cartesian Transformation/3(RawX) -> Mux/1
  Jacobian-Cartesian Transformation/4(RawY) -> Mux/2
  [Reward] -> For Iterator Subsystem/3(Reward)
  Jacobian-Cartesian Transformation/5(Jacobian) -> J/1
  Mux/1 -> RawPos/1
  [Word] -> For Iterator Subsystem/4(Word)
  Mux2/1 -> Th/1
  Cursor Rotation1/1(Xo) -> Mux3/1
  Cursor Rotation1/2(Yo) -> Mux3/2
  PCI-6025E AD/1 -> Mux4/1
  PCI-6025E AD/2 -> Mux4/2
  PCI-6025E AD/3 -> Mux4/3
  PCI-6025E AD/4 -> Mux4/4
  PCI-6025E AD/5 -> Mux4/5
  PCI-6025E AD/6 -> Mux4/6
  Dot Product X/1 -> Avg/1(In)
  Add/1 -> Cursor Rotation1/1(Xi)
  Dot Product Y/1 -> Avg1/1(In)
  Add1/1 -> Cursor Rotation1/2(Yi)
  Demux/1 -> Add/1
  Demux/2 -> Add1/1
  Mux4/1 -> Add2/1, OffsetCalculation/1(RawForce)
  Add2/1 -> Dot Product Y/1, Dot Product X/1
  Avg/1(Out) -> Handle Rotation/1(Xin)
  Avg1/1(Out) -> Handle Rotation/2(Yin)
  Handle Rotation/2(Yout) -> Dot Product1/1
  [Offsets] -> Demux/1
  Mux3/1 -> Switch/1
  Switch/1 -> Pos/1
  Mux1/1 -> Switch/3
  IsometricMode/1 -> Switch/2
  Dot Product/1 -> Add/2
  UpsideDownHandle/1 -> Fcn/1
  Fcn/1 -> Dot Product/1
  LoadCellXCoef1/1 -> Vector Concatenate/1
  LoadCellXCoef2/1 -> Vector Concatenate/2
  LoadCellXCoef3/1 -> Vector Concatenate/3
  LoadCellXCoef4/1 -> Vector Concatenate/4
  LoadCellXCoef5/1 -> Vector Concatenate/5
  LoadCellXCoef6/1 -> Vector Concatenate/6
  LoadCellYCoef1/1 -> Vector Concatenate1/1
  LoadCellYCoef2/1 -> Vector Concatenate1/2
  LoadCellYCoef3/1 -> Vector Concatenate1/3
  LoadCellYCoef4/1 -> Vector Concatenate1/4
  LoadCellYCoef5/1 -> Vector Concatenate1/5
  LoadCellYCoef6/1 -> Vector Concatenate1/6
  Vector Concatenate/1 -> Gain2/1
  Vector Concatenate1/1 -> Gain3/1
  Dot Product1/1 -> Add1/2
  Dot Product2/1 -> Dot Product/2
  Handle Rotation/1(Xout) -> Dot Product2/1
  ForceToScreenGain/1 -> Dot Product1/2, Dot Product2/2
  Gain2/1 -> Dot Product X/2
  Gain3/1 -> Dot Product Y/2
  OffsetCalculation/1(Offsets) -> Add2/2
  Compare To Constant/1 -> Switch1/2
  LabNumber/1 -> Compare To Constant/1
  Switch1/1 -> Handle Rotation/3(ElbowAngle)

== system limblab/Force Generator/LorentzForce ==
  Add : Sum  Inputs=+-
  Add1 : Sum  Inputs=+-
  Lorentz : limblab/Lorentz  y0=.1
  Lorentz1 : limblab/Lorentz  y0=.2
  Lorentz2 : limblab/Lorentz  y0=.3
  Lorentz3 : limblab/Lorentz  y0=.4
  X : Outport
  Y : Outport  Port=2
  wires:
  Lorentz/1 -> Add/1
  Lorentz1/1 -> Add/2
  Add/1 -> X/1
  Lorentz2/1 -> Add1/1
  Lorentz3/1 -> Add1/2
  Add1/1 -> Y/1

== system limblab/Force Generator/ViscLoadSubsystem ==
  Vel : Inport
  Angle : Inport  Port=2
  Add : Sum
  Demux : Demux  Outputs=2
  Gain : Gain
  Inverter : Gain  Gain=-1
  Mux : Mux  Inputs=2
  Product{,1..3} (4 alike) : Product  RndMeth=Zero
  Subtract : Sum  Inputs=+-
  cos : Trigonometry  Operator=cos
  sin : Trigonometry
  LoadOut : Outport
  wires:
  Mux/1 -> Gain/1
  Angle/1 -> sin/1, cos/1
  Add/1 -> Mux/1
  Subtract/1 -> Mux/2
  Product/1 -> Add/1
  Product1/1 -> Add/2
  Product2/1 -> Subtract/1
  Product3/1 -> Subtract/2
  Demux/1 -> Product/1, Product3/1
  cos/1 -> Product/2, Product2/2
  Demux/2 -> Product1/1, Product2/1
  sin/1 -> Product1/2, Product3/2
  Gain/1 -> LoadOut/1
  Vel/1 -> Inverter/1
  Inverter/1 -> Demux/1

== system limblab/Motor Control/Force/Torque Transform ==
  F : Inport
  J : Inport  Port=2
  Demux2 : Demux  Outputs=2
  Gain : Gain  Gain=-1
  Matrix Multiply : Product  Multiplication=Matrix(*)
  Transpose : dspmtrx3/Transpose  Hermitian=off  overflowFlag=off
  T1 : Outport
  T2 : Outport  Port=2
  wires:
  J/1 -> Transpose/1
  Transpose/1 -> Matrix Multiply/1
  Matrix Multiply/1 -> Demux2/1
  Demux2/2 -> T2/1
  Demux2/1 -> T1/1
  Gain/1 -> Matrix Multiply/2
  F/1 -> Gain/1

== system limblab/Motor Control/Schmidt ==
  In1 : Inport
  Clock : Clock
  Compare To Zero : simulink/Logic and Bit Operations/Compare To Zero  relop=>  OutDataTypeStr=uint8  ZeroCross=off
  Enabled Subsystem : Subsystem  TreatAsAtomicUnit=on
  Logical Operator : Logic  Operator=XOR  AllPortsSameDT=off  OutDataTypeStr=boolean  SampleTime=.001
  Logical Operator1 : Logic  Operator=NOT  AllPortsSameDT=off  OutDataTypeStr=boolean
  Logical Operator2 : Logic  Operator=OR  AllPortsSameDT=off  OutDataTypeStr=boolean  SampleTime=.001
  Memory : Memory
  Relational Operator : RelationalOperator  Operator=>  OutDataTypeStr=boolean
  Sum : Sum  Inputs=-+
  Time : Constant  Value=Time
  Out1 : Outport
  wires:
  Clock/1 -> Enabled Subsystem/1(In1), Sum/2
  Enabled Subsystem/1(Out1) -> Sum/1
  Sum/1 -> Compare To Zero/1, Relational Operator/1
  Time/1 -> Relational Operator/2
  Compare To Zero/1 -> Logical Operator/1
  Relational Operator/1 -> Logical Operator/2
  Logical Operator1/1 -> Enabled Subsystem/Enable
  Logical Operator/1 -> Out1/1, Memory/1
  In1/1 -> Logical Operator2/2
  Logical Operator2/1 -> Logical Operator1/1
  Memory/1 -> Logical Operator2/1

== system limblab/Recentering Subsystem/No Movement ==
  Vel : Inport
  Abs2 : Abs
  Abs3 : Abs
  Compare To Constant2 : simulink/Logic and Bit Operations/Compare To Constant  relop=<=  const=0.004  OutDataTypeStr=uint8  ZeroCross=off
  Compare To Constant3 : simulink/Logic and Bit Operations/Compare To Constant  relop=<=  const=.004  OutDataTypeStr=uint8  ZeroCross=off
  Demux1 : Demux  Outputs=2
  Logical Operator1 : Logic  AllPortsSameDT=off  OutDataTypeStr=boolean
  NotMoving : Outport
  wires:
  Abs2/1 -> Compare To Constant2/1
  Abs3/1 -> Compare To Constant3/1
  Logical Operator1/1 -> NotMoving/1
  Vel/1 -> Demux1/1
  Demux1/1 -> Abs2/1
  Demux1/2 -> Abs3/1
  Compare To Constant2/1 -> Logical Operator1/1
  Compare To Constant3/1 -> Logical Operator1/2

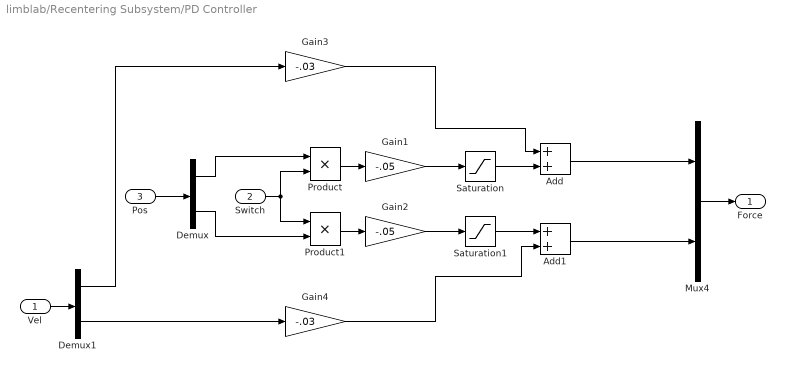
== system limblab/Recentering Subsystem/PD Controller ==
  Vel : Inport
  Switch : Inport  Port=2
  Pos : Inport  Port=3
  Add : Sum
  Add1 : Sum
  Demux : Demux  Outputs=2
  Demux1 : Demux  Outputs=2
  Gain1 : Gain  Gain=-.05
  Gain2 : Gain  Gain=-.05
  Gain3 : Gain  Gain=-.03
  Gain4 : Gain  Gain=-.03
  Mux4 : Mux  Inputs=2
  Product : Product  RndMeth=Zero
  Product1 : Product  RndMeth=Zero
  Saturation : Saturate  UpperLimit=3  LowerLimit=-3
  Saturation1 : Saturate  UpperLimit=3  LowerLimit=-3
  Force : Outport
  wires:
  Switch/1 -> Product/2, Product1/1
  Product/1 -> Gain1/1
  Add/1 -> Mux4/1
  Gain1/1 -> Saturation/1
  Gain3/1 -> Add/1
  Product1/1 -> Gain2/1
  Add1/1 -> Mux4/2
  Gain2/1 -> Saturation1/1
  Gain4/1 -> Add1/2
  Mux4/1 -> Force/1
  Demux/1 -> Product/1
  Demux/2 -> Product1/2
  Pos/1 -> Demux/1
  Vel/1 -> Demux1/1
  Demux1/2 -> Gain4/1
  Demux1/1 -> Gain3/1
  Saturation/1 -> Add/2
  Saturation1/1 -> Add1/1

== system limblab/Recentering Subsystem/Schmidt1 ==
  In1 : Inport
  Clock : Clock
  Compare To Zero : simulink/Logic and Bit Operations/Compare To Zero  relop=>  OutDataTypeStr=uint8  ZeroCross=off
  Enabled Subsystem : Subsystem  TreatAsAtomicUnit=on
  Logical Operator : Logic  Operator=XOR  AllPortsSameDT=off  OutDataTypeStr=boolean  SampleTime=.001
  Logical Operator1 : Logic  Operator=NOT  AllPortsSameDT=off  OutDataTypeStr=boolean
  Logical Operator2 : Logic  Operator=OR  AllPortsSameDT=off  OutDataTypeStr=boolean  SampleTime=.001
  Memory : Memory
  Relational Operator : RelationalOperator  Operator=>  OutDataTypeStr=boolean
  Sum : Sum  Inputs=-+
  Time : Constant  Value=Time
  Out1 : Outport
  wires:
  Clock/1 -> Enabled Subsystem/1(In1), Sum/2
  Enabled Subsystem/1(Out1) -> Sum/1
  Sum/1 -> Compare To Zero/1, Relational Operator/1
  Time/1 -> Relational Operator/2
  Compare To Zero/1 -> Logical Operator/1
  Relational Operator/1 -> Logical Operator/2
  Logical Operator1/1 -> Enabled Subsystem/Enable
  Logical Operator/1 -> Out1/1, Memory/1
  In1/1 -> Logical Operator2/2
  Logical Operator2/1 -> Logical Operator1/1
  Memory/1 -> Logical Operator2/1

== system limblab/Recentering Subsystem/Schmidt2 ==
  In1 : Inport
  Clock : Clock
  Compare To Zero : simulink/Logic and Bit Operations/Compare To Zero  relop=>  OutDataTypeStr=uint8  ZeroCross=off
  Enabled Subsystem : Subsystem  TreatAsAtomicUnit=on
  Logical Operator : Logic  Operator=XOR  AllPortsSameDT=off  OutDataTypeStr=boolean  SampleTime=.001
  Logical Operator1 : Logic  Operator=NOT  AllPortsSameDT=off  OutDataTypeStr=boolean
  Logical Operator2 : Logic  Operator=OR  AllPortsSameDT=off  OutDataTypeStr=boolean  SampleTime=.001
  Memory : Memory
  Relational Operator : RelationalOperator  Operator=>  OutDataTypeStr=boolean
  Sum : Sum  Inputs=-+
  Time : Constant  Value=Time
  Out1 : Outport
  wires:
  Clock/1 -> Enabled Subsystem/1(In1), Sum/2
  Enabled Subsystem/1(Out1) -> Sum/1
  Sum/1 -> Compare To Zero/1, Relational Operator/1
  Time/1 -> Relational Operator/2
  Compare To Zero/1 -> Logical Operator/1
  Relational Operator/1 -> Logical Operator/2
  Logical Operator1/1 -> Enabled Subsystem/Enable
  Logical Operator/1 -> Out1/1, Memory/1
  In1/1 -> Logical Operator2/2
  Logical Operator2/1 -> Logical Operator1/1
  Memory/1 -> Logical Operator2/1

== system limblab/Recentering Subsystem/Schmidt3 ==
  In1 : Inport
  Clock : Clock
  Compare To Zero : simulink/Logic and Bit Operations/Compare To Zero  relop=>  OutDataTypeStr=uint8  ZeroCross=off
  Enabled Subsystem : Subsystem  TreatAsAtomicUnit=on
  Logical Operator : Logic  Operator=XOR  AllPortsSameDT=off  OutDataTypeStr=boolean  SampleTime=.001
  Logical Operator1 : Logic  Operator=NOT  AllPortsSameDT=off  OutDataTypeStr=boolean
  Logical Operator2 : Logic  Operator=OR  AllPortsSameDT=off  OutDataTypeStr=boolean  SampleTime=.001
  Memory : Memory
  Relational Operator : RelationalOperator  Operator=>  OutDataTypeStr=boolean
  Sum : Sum  Inputs=-+
  Time : Constant  Value=Time
  Out1 : Outport
  wires:
  Clock/1 -> Enabled Subsystem/1(In1), Sum/2
  Enabled Subsystem/1(Out1) -> Sum/1
  Sum/1 -> Compare To Zero/1, Relational Operator/1
  Time/1 -> Relational Operator/2
  Compare To Zero/1 -> Logical Operator/1
  Relational Operator/1 -> Logical Operator/2
  Logical Operator1/1 -> Enabled Subsystem/Enable
  Logical Operator/1 -> Out1/1, Memory/1
  In1/1 -> Logical Operator2/2
  Logical Operator2/1 -> Logical Operator1/1
  Memory/1 -> Logical Operator2/1

== system limblab/ResetableSchmidt/Enabled Subsystem ==
  In1 : Inport
  Enable : EnablePort
  Out1 : Outport
  wires:
  In1/1 -> Out1/1

== system limblab/RewardSbs/Schmidt ==
  Trigger : Inport
  Duration : Inport  Port=2
  Clock : Clock
  Relational Operator : RelationalOperator  Operator=<  OutDataTypeStr=boolean
  Sample and Hold : dspsigops/Sample and Hold  trig=Rising edge  initCond=-1000  latchinput=off
  Sum : Sum  Inputs=-+
  Output : Outport
  wires:
  Clock/1 -> Sum/2, Sample and Hold/1
  Sample and Hold/1 -> Sum/1
  Sum/1 -> Relational Operator/1
  Duration/1 -> Relational Operator/2
  Relational Operator/1 -> Output/1
  Trigger/1 -> Sample and Hold/Trigger

== system limblab/Schmidt/Enabled Subsystem ==
  In1 : Inport
  Enable : EnablePort
  Out1 : Outport
  wires:
  In1/1 -> Out1/1

== system limblab/Velocity Calculation/Pos2VelX ==
  In : Inport
  Derivative : Derivative
  Digital Filter : dsparch4/Digital Filter  TypePopup=FIR (all zeros)  IIRFiltStruct=Direct form II transposed  AllPoleFiltStruct=Direct form  FIRFiltStruct=Direct form  CoeffSource=Specify via dialog  NumCoeffs="[0.0144    0.0304    0.0724    0.1245    0.1668    0.1830    0.1668    0.1245    0.0724    0.0304    0.0144]"  DenCoeffs=[1 0.1]  BiQuadCoeffs=[1 0.3 0.4 1 0.1 0.2]  LatticeCoeffs=[0.2 0.4]  denIgnore=on  FiltPerSampPopup=One filter per frame  IC=0  ICnum=0  ICden=0  roundingMode=Floor  overflowMode=off  ScaleValues=1  scaleValueFracLength=14  stageInFracLength=15  stageOutFracLength=15  FilterSource=Specify via dialog  dfiltObjectName=dfilt.dffir([1 2 1])  InputProcessing=Inherited (this choice will be removed - see release notes)
  Digital Filter2 : dsparch4/Digital Filter  TypePopup=FIR (all zeros)  IIRFiltStruct=Direct form II transposed  AllPoleFiltStruct=Direct form  FIRFiltStruct=Direct form  CoeffSource=Specify via dialog  NumCoeffs="[0.0144    0.0304    0.0724    0.1245    0.1668    0.1830    0.1668    0.1245    0.0724    0.0304    0.0144]"  DenCoeffs=[1 0.1]  BiQuadCoeffs=[1 0.3 0.4 1 0.1 0.2]  LatticeCoeffs=[0.2 0.4]  denIgnore=on  FiltPerSampPopup=One filter per frame  IC=0  ICnum=0  ICden=0  roundingMode=Floor  overflowMode=off  ScaleValues=1  scaleValueFracLength=14  stageInFracLength=15  stageOutFracLength=15  FilterSource=Specify via dialog  dfiltObjectName=dfilt.dffir([1 2 1])  InputProcessing=Inherited (this choice will be removed - see release notes)
  dG : Gain  SampleTime=.001
  Out : Outport
  wires:
  Derivative/1 -> dG/1
  dG/1 -> Digital Filter/1
  Digital Filter2/1 -> Derivative/1
  In/1 -> Digital Filter2/1
  Digital Filter/1 -> Out/1

== system limblab/Velocity Calculation/Pos2VelY ==
  In : Inport
  Derivative : Derivative
  Digital Filter : dsparch4/Digital Filter  TypePopup=FIR (all zeros)  IIRFiltStruct=Direct form II transposed  AllPoleFiltStruct=Direct form  FIRFiltStruct=Direct form  CoeffSource=Specify via dialog  NumCoeffs="[0.0144    0.0304    0.0724    0.1245    0.1668    0.1830    0.1668    0.1245    0.0724    0.0304    0.0144]"  DenCoeffs=[1 0.1]  BiQuadCoeffs=[1 0.3 0.4 1 0.1 0.2]  LatticeCoeffs=[0.2 0.4]  denIgnore=on  FiltPerSampPopup=One filter per frame  IC=0  ICnum=0  ICden=0  roundingMode=Floor  overflowMode=off  ScaleValues=1  scaleValueFracLength=14  stageInFracLength=15  stageOutFracLength=15  FilterSource=Specify via dialog  dfiltObjectName=dfilt.dffir([1 2 1])  InputProcessing=Inherited (this choice will be removed - see release notes)
  Digital Filter2 : dsparch4/Digital Filter  TypePopup=FIR (all zeros)  IIRFiltStruct=Direct form II transposed  AllPoleFiltStruct=Direct form  FIRFiltStruct=Direct form  CoeffSource=Specify via dialog  NumCoeffs="[0.0144    0.0304    0.0724    0.1245    0.1668    0.1830    0.1668    0.1245    0.0724    0.0304    0.0144]"  DenCoeffs=[1 0.1]  BiQuadCoeffs=[1 0.3 0.4 1 0.1 0.2]  LatticeCoeffs=[0.2 0.4]  denIgnore=on  FiltPerSampPopup=One filter per frame  IC=0  ICnum=0  ICden=0  roundingMode=Floor  overflowMode=off  ScaleValues=1  scaleValueFracLength=14  stageInFracLength=15  stageOutFracLength=15  FilterSource=Specify via dialog  dfiltObjectName=dfilt.dffir([1 2 1])  InputProcessing=Inherited (this choice will be removed - see release notes)
  dG : Gain  SampleTime=.001
  Out : Outport
  wires:
  Derivative/1 -> dG/1
  dG/1 -> Digital Filter/1
  Digital Filter2/1 -> Derivative/1
  In/1 -> Digital Filter2/1
  Digital Filter/1 -> Out/1

== system limblab/XY Position Subsystem/Avg ==
  In : Inport
  Gain : Gain  Gain=16
  Gain1 : Gain  Gain=1/17
  Sum : Sum  Inputs=|++
  Unit Delay : UnitDelay  SampleTime=.001
  Out : Outport
  wires:
  In/1 -> Sum/1
  Gain/1 -> Sum/2
  Unit Delay/1 -> Gain/1
  Sum/1 -> Gain1/1
  Gain1/1 -> Out/1, Unit Delay/1

== system limblab/XY Position Subsystem/Avg1 ==
  In : Inport
  Gain : Gain  Gain=16
  Gain1 : Gain  Gain=1/17
  Sum : Sum  Inputs=|++
  Unit Delay : UnitDelay  SampleTime=.001
  Out : Outport
  wires:
  In/1 -> Sum/1
  Gain/1 -> Sum/2
  Unit Delay/1 -> Gain/1
  Sum/1 -> Gain1/1
  Gain1/1 -> Out/1, Unit Delay/1

== system limblab/XY Position Subsystem/Cursor Rotation ==
  Xi : Inport
  Yi : Inport  Port=2
  AngleOffset : Constant  Value=0  SampleTime=.001
  Mux : Mux  Inputs=2
  Product : Product  RndMeth=Zero
  Product1 : Product  RndMeth=Zero
  Sum : Sum  Inputs=|++
  Trigonometric Function : Trigonometry
  Trigonometric Function1 : Trigonometry  Operator=atan2
  Trigonometric Function2 : Trigonometry  Operator=cos
  sqrt(u[1]*u[1] + u[2]*u[2]) : Fcn  Expr=sqrt(u[1]*u[1] + u[2]*u[2])
  Xo : Outport
  Yo : Outport  Port=2
  wires:
  AngleOffset/1 -> Sum/2
  Trigonometric Function1/1 -> Sum/1
  Yi/1 -> Trigonometric Function1/1, Mux/1
  Xi/1 -> Trigonometric Function1/2, Mux/2
  Mux/1 -> sqrt(u[1]*u[1] + u[2]*u[2])/1
  Trigonometric Function/1 -> Product/2
  Product/1 -> Yo/1
  sqrt(u[1]*u[1] + u[2]*u[2])/1 -> Product/1, Product1/2
  Sum/1 -> Trigonometric Function/1, Trigonometric Function2/1
  Product1/1 -> Xo/1
  Trigonometric Function2/1 -> Product1/1

== system limblab/XY Position Subsystem/Cursor Rotation1 ==
  Xi : Inport
  Yi : Inport  Port=2
  AngleOffset : Constant  Value=0  SampleTime=.001
  Mux : Mux  Inputs=2
  Product : Product  RndMeth=Zero
  Product1 : Product  RndMeth=Zero
  Sum : Sum  Inputs=|++
  Trigonometric Function : Trigonometry
  Trigonometric Function1 : Trigonometry  Operator=atan2
  Trigonometric Function2 : Trigonometry  Operator=cos
  sqrt(u[1]*u[1] + u[2]*u[2]) : Fcn  Expr=sqrt(u[1]*u[1] + u[2]*u[2])
  Xo : Outport
  Yo : Outport  Port=2
  wires:
  AngleOffset/1 -> Sum/2
  Trigonometric Function1/1 -> Sum/1
  Yi/1 -> Trigonometric Function1/1, Mux/1
  Xi/1 -> Trigonometric Function1/2, Mux/2
  Mux/1 -> sqrt(u[1]*u[1] + u[2]*u[2])/1
  Trigonometric Function/1 -> Product/2
  Product/1 -> Yo/1
  sqrt(u[1]*u[1] + u[2]*u[2])/1 -> Product/1, Product1/2
  Sum/1 -> Trigonometric Function/1, Trigonometric Function2/1
  Product1/1 -> Xo/1
  Trigonometric Function2/1 -> Product1/1
